simulink model "SwarmSystem"  (R2022b)
settings: Solver=VariableStepAuto  StartTime=0.0  StopTime=10.0  RelTol=1e-3
values from neighbouring files (symbols this model uses):
  dt = 0.01    [init_params.m]
  initial_state_x0 = Simulink.Parameter(initial_state_x0)    [init_params.m]    (also in single_model_verification_script.m = [W0; R0; dP0; P0]; team_model_conf_comp_script.m = [W0; R0; dP0; P0]; team_model_tethered_tilt.m = [W0; R0; dP0; P0]; team_model_tracking_script.m = [W0; R0; dP0; P0])
undefined symbols (not defined in the file or in its folder): drone_params, env_params
libraries: dspindex x15, aerolibanim x1
(part 4 of 4)

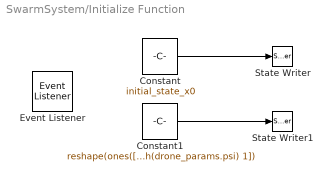
== system SwarmSystem/Initialize Function ==
  Constant : Constant  Value=initial_state_x0  VectorParams1D=off
  Constant1 : Constant  Value=reshape(ones([1 length(drone_params.psi)]) .* [0 0 0 0 1 1]', [6*length(drone_params.psi) 1])  VectorParams1D=off
  Event Listener : EventListener  DisableCoverage=on  EventName=reset
  State Writer : StateWriter  StateOwnerBlock=../../DroneState
  State Writer1 : StateWriter  StateOwnerBlock=../../InternalState
  wires:
  Constant/1 -> State Writer/1
  Constant1/1 -> State Writer1/1

== matlab function SwarmSystem/MATLAB Function3 ==
  data: R input; eulers output
function eulers = rotm2euler(R)
    psi = atan2(-R(1, 2), R(2, 2));    
    phi = atan2(R(3, 2), sqrt(abs(1-R(3, 2).^2)));
    theta = atan2(-R(3, 1), R(3, 3));
    eulers = [psi phi theta]';
end

== matlab function SwarmSystem/MATLAB Function5 ==
  data: zo input; drone_params parameter; vec output; env_params parameter
function vec = actuator_mixing(zo, drone_params, env_params)
    %% Parameters
    g = env_params.g; % gravity
    rho = env_params.rho; % kg/m3
    prop_d = env_params.prop_d; % 8 inch = 20.3 cm
    
    CT_u = env_params.CT_u; % upper propeller thrust coefficient
    CT_l = env_params.CT_l; % lower propeller thrust coefficient
    CP_u = env_params.CP_u; % upper propeller drag coefficient
    CP_l = env_params.CP_l; % lower propeller drag coefficient

    pos = drone_params.pos;
    psi = drone_params.psi;
    n = length(psi);

    Tf = zeros([n 1]);
    eta_x = zeros([n 1]);
    eta_y = zeros([n 1]);

    beta_allo = [CT_u CT_l; prop_d * CP_u -prop_d * CP_l];
    P_prop = rho * prop_d^4 * beta_allo;

    for i = 1:n
        % Actuator Model
        zi = zo(4 * (i - 1) + 1 : 4 * i);
        TfTdi = P_prop * zi(3:4, 1).^2;
        Tf(i) = TfTdi(1);
        eta_x(i) = zi(1);
        eta_y(i) = zi(2);
    end

    M = get_M(n, psi, pos);
    fi = get_f(eta_x, eta_y, Tf);
    vec = M * fi;
end

== matlab function SwarmSystem/MATLAB Function6 ==
  data: zo input; drone_params parameter; vec output; env_params parameter
function vec = actuator_mixing(zo, drone_params, env_params)
    %% Parameters
    g = env_params.g; % gravity
    rho = env_params.rho; % kg/m3
    prop_d = env_params.prop_d; % 8 inch = 20.3 cm
    
    CT_u = env_params.CT_u; % upper propeller thrust coefficient
    CT_l = env_params.CT_l; % lower propeller thrust coefficient
    CP_u = env_params.CP_u; % upper propeller drag coefficient
    CP_l = env_params.CP_l; % lower propeller drag coefficient

    pos = drone_params.pos;
    psi = drone_params.psi;
    n = length(psi);

    Tf = zeros([n 1]);
    eta_x = zeros([n 1]);
    eta_y = zeros([n 1]);

    beta_allo = [CT_u CT_l; prop_d * CP_u -prop_d * CP_l];
    P_prop = rho * prop_d^4 * beta_allo;

    for i = 1:n
        % Actuator Model
        zi = zo(4 * (i - 1) + 1 : 4 * i);
        TfTdi = P_prop * zi(3:4, 1).^2;
        Tf(i) = TfTdi(1);
        eta_x(i) = zi(1);
        eta_y(i) = zi(2);
    end

    M = get_M(n, psi, pos);
    fi = get_f(eta_x, eta_y, Tf);
    vec = M * fi;
end

== matlab function SwarmSystem/Actuator Compensator ==
  settings: updateMethod=DISCRETE  sampleTime=dt
  data: z input; z_d input; z_dc output; drone_params parameter; dt parameter
function z_dc = acutator_compensator(z, z_d, drone_params, dt)
    psi = drone_params.psi;
    n = length(psi);    
    
    mKp = drone_params.mKp; % Servo motor gain
    mKd = drone_params.mKd; % Servo motor gain
    pKp = drone_params.pKp; % BLDC motor gain

    sigma_x = drone_params.sigma_a;
    sigma_y = drone_params.sigma_b;
    z_dc = opt_compensator(n, z, z_d, sigma_x, sigma_y);
    %z_dc = compensator(n, z, z_d, dt, mKp, mKd, sigma_x, sigma_y);
end

function z_dc = opt_compensator(n, z, z_d, sigma_x, sigma_y)
    z_dc = z_d;
    for i=1:n
        zi = z(6*(i-1)+1 : 6*i);
        x_zi = [1 0 0 0 0 0; 0 0 1 0 0 0] * zi;
        v_zi = [0 1 0 0 0 0; 0 0 0 1 0 0] * zi;

        z_di = z_d(4*(i-1)+1 : 4*(i-1)+2);
        %z_dcr = -14.3636 * (x_zi-z_di) - 0.3070 * (v_zi-0) + 0.6924 * z_di;
        z_dcr = -28.0209 * (x_zi-z_di) -0.5379 * (v_zi-0) + 0.9971 * z_di;
        %z_dcr = -17.3915 * (x_zi-z_di) -0.4492 * (v_zi-0) + 0.8054 * z_di;
        %z_dcr = -11.8288 * (x_zi-z_di) -0.4958 * (v_zi-0) + 0.4905 * z_di;
        
        z_dcr(1) = min(sigma_x, max(-sigma_x, z_dcr(1)));
        z_dcr(2) = min(sigma_y, max(-sigma_y, z_dcr(2)));

        z_dc(4*(i-1)+1 : 4*(i-1)+2) = z_dcr;
    end
end

function z_dc = compensator(n, z, z_d, dt, mKp, mKd, sigma_x, sigma_y)
    w_n = sqrt(mKp);
    zeta = mKd / (2 * w_n);
    k = mKp;

    w_d = w_n * sqrt(1 - zeta^2);
    sigma = -zeta * w_n;

    C1 = (w_n / w_d) * exp(sigma * dt) * sin(w_d * dt + atan(w_d / -sigma));
    C2 = (exp(sigma * dt) / w_d) * sin(w_d * dt);
    C3 = (k / w_d) * (w_d + exp(sigma * dt) * (sigma*sin(w_d*dt) - w_d*cos(w_d*dt))) / w_n^2;

    z_dc = z_d;
    %return
    
    for i=1:n
        zi = z(6*(i-1)+1 : 6*i);
        x_zi = [1 0 0 0 0 0; 0 0 1 0 0 0] * zi;
        v_zi = [0 1 0 0 0 0; 0 0 0 1 0 0] * zi;

        z_di = z_d(4*(i-1)+1 : 4*(i-1)+2);
        delta_z_di = z_di - x_zi;

        M = (delta_z_di + (1-C3-C1)*x_zi - C2*v_zi) ./ (C3 * delta_z_di);
        z_dcr = x_zi + delta_z_di .* M;
        
        z_dcr(1) = min(sigma_x, max(-sigma_x, z_dcr(1)));
        z_dcr(2) = min(sigma_y, max(-sigma_y, z_dcr(2)));

        z_dc(4*(i-1)+1 : 4*(i-1)+2) = z_dcr;
    end
end

== matlab function SwarmSystem/MATLAB Function7 ==
  data: u input; alignment output; u_d input; error output
function [alignment, error] = metrices(u, u_d)
    error = norm(u_d - u) / norm(u_d);
    alignment = u' * u_d / (norm(u_d) * norm(u));
end

== matlab function SwarmSystem/MATLAB Function8 ==
  data: u input; alignment output; u_d input; error output
function [alignment, error] = metrices(u, u_d)
    error = norm(u_d - u) / norm(u_d);
    alignment = u' * u_d / (norm(u_d) * norm(u));
end

== matlab function SwarmSystem/Full-Pose Controller ==
  settings: updateMethod=DISCRETE  sampleTime=dt
  data: x_r input; u_d output size=[6 1]; R_r input; x input; env_params parameter; drone_params parameter; R_d output
function [u_d, R_d] = full_pose_controller(x_r, R_r, x, env_params, drone_params)
    m = drone_params.m; % Mass, Kg
    g = env_params.g;
    I_b = drone_params.I_b; % Leverage length from c.p. to c.g.
    
    % States
    p = x(16:18);
    v = x(13:15);
    R = reshape(x(4:12), [3 3]); % 3x3
    w = x(1:3);
    
    % Gain
    Kp = diag([1 1 1]) * 0.2 * 10;
    Kd = diag([1 1 1]) * 0.5 * 10;
    Kr = diag([1 1 1]) * 3 * 10;
    Ko = diag([1 1 1]) * 1 * 10;
    
    % % Translational error
    ep = p - x_r(1:3, 1);
    ev = v - x_r(1:3, 2);
    
    f_r = m * x_r(1:3, 3) + m*[0; 0; g] + m * (- Kp * ep - Kd * ev);
    u_f = R' * f_r;
    u_f = force_sat(drone_params, u_f);
    
    [R_d, theta] = calc_R_d(drone_params, f_r, R_r);
    %R_d = R_r;
    % w_d = vee(R_d' * d_R_d);
    
    % Attitude error
    eRx = 0.5 * (R_d' * R - R' * R_d);
    eR = vee(eRx);
    % eOmega = w - R' * R_d * w_d;
    eOmega = w;
    
    u_tau = cross(w, I_b * w) + I_b * ( - Kr * eR - Ko * eOmega);
    u_d = [u_f; u_tau];
end

function u_sat = force_sat(drone_params, u)
    psi = drone_params.psi;
    sigma_a = drone_params.sigma_a;
    f_max = drone_params.f_max;
    n = length(psi);

    n_x = sum(psi == 0);
    n_y = n - n_x;

    a = n_x * f_max + (n_y ~= 0) * u(3) * tan(sigma_a);
    b = n_y * f_max + (n_x ~= 0) * u(3) * tan(sigma_a);
    t = (a * b) / sqrt(u(1)^2 * b^2 + u(2)^2 * a^2);

    % Directional saturation
    u_sat = u;
    if t < 1
        u_sat(1:2) = t * u(1:2);
    end

    % Magnitude saturation
    roof_lim = n * drone_params.f_max;
    scale = norm(u_sat(1:3)) / roof_lim;
    if scale > 1
        u_sat(1:3) = u_sat(1:3) / scale;
    end
end

function [R_d, theta] = calc_R_d(drone_params, f_r, R_r)
    b1r = R_r(:, 1);
    b2r = R_r(:, 2);
    b3r = R_r(:, 3);
    [theta] = ctrl_sat_square_bisection(drone_params, 20, b1r, b3r, f_r);

    k = cross(b3r, f_r) / norm(cross(b3r, f_r));
    nb3 = rot_vec_by_theta(b3r, k, theta);
    nb2 = cross(nb3, b1r) / norm(cross(nb3, b1r));
    nb1 = cross(nb2, nb3);
    R_d = [nb1 nb2 nb3];
end

function [theta] = ctrl_sat_square_bisection(drone_params, n, b1r, b3r, f_r)
    %sigma_a = conf('sigma_a');
    b2r = cross(b3r, b1r);
    theta_max = acos(b3r' * f_r / norm(f_r));
    % theta_max = asin(norm(cross(b3r, f_r)) / norm(f_r));
    theta = theta_max / 2;
    % abs(f_r' * b2r)
    % f_r' * b3r * tan(sigma_a)
    % if abs(f_r' * b2r) > f_r' * b3r * tan(sigma_a)
    if ~is_attainable(drone_params, b1r, b2r, b3r, f_r)
        k = cross(b3r, f_r) / norm(cross(b3r, f_r));
        for i=1:n
            b3 = rot_vec_by_theta(b3r, k, theta);
            b2 = cross(b3, b1r) / norm(cross(b3, b1r));
            b1 = cross(b2, b3);
            % if abs(f_r' * b2) < f_r' * b3 * tan(sigma_a)
            if is_attainable(drone_params, b1, b2, b3, f_r)
                theta = theta - 0.5 * theta_max / (2^i);
            else
                theta = theta + 0.5 * theta_max / (2^i);
            end
            % fprintf("%d: %.4f\n", i, theta)
        end
    else
        theta = 0;
    end
end

function out = rot_vec_by_theta(vec, rot_axis, theta)
    out = vec * cos(theta) + cross(rot_axis, vec) * sin(theta) + rot_axis * (rot_axis' * vec) * (1 - cos(theta));
end

function feasible = is_attainable(drone_params, b1, b2, b3, f_r)
    feasible = elliptic_cone(drone_params, b1, b2, b3, f_r);
    % feasible = pie(conf, b1, b2, b3, f_r);
end

function feasible = elliptic_cone(drone_params, b1, b2, b3, f_r)
    n = length(drone_params.psi);
    f_max = drone_params.f_max;
    sigma_a = drone_params.sigma_a;
    sigma_b = drone_params.sigma_b;

    n_x = sum(drone_params.psi == 0);
    n_y = n - n_x;

    z = f_r' * b3;
    c_x = fun_g(n_x, sigma_b, z, f_max) + fun_g(n_y, sigma_a, z, f_max);
    c_y = fun_g(n_x, sigma_a, z, f_max) + fun_g(n_y, sigma_b, z, f_max);

    feasible = (z > 0) & (((f_r' * b1 / c_x)^2 + (f_r' * b2 / c_y)^2) <= 1);
end

function gk = fun_g(n_k, sigma_k_bar, z, f_max)
    if (sigma_k_bar >= pi / 2)
        gk = n_k * f_max;
    else
        gk = (n_k > 0) * z * tan(sigma_k_bar);
    end
end

== matlab function SwarmSystem/SwarmModel ==
  data: x input; z input; dxdt output; z_d input; dzdt output; env_params parameter; drone_params parameter
function [dxdt, dzdt] = swarm_model(x, z, z_d, env_params, drone_params)
    %% Parameters
    g = env_params.g; % gravity
    rho = env_params.rho; % kg/m3
    prop_d = env_params.prop_d; % 8 inch = 20.3 cm
    
    CT_u = env_params.CT_u; % upper propeller thrust coefficient
    CT_l = env_params.CT_l; % lower propeller thrust coefficient
    CP_u = env_params.CP_u; % upper propeller drag coefficient
    CP_l = env_params.CP_l; % lower propeller drag coefficient
    
    mKp = drone_params.mKp; % Servo motor gain
    mKd = drone_params.mKd; % Servo motor gain
    pKp = drone_params.pKp; % BLDC motor gain
    
    % Bounds
    sigma_x = drone_params.sigma_a;
    sigma_y = drone_params.sigma_b;
    r_sigma_x = drone_params.r_sigma_a;
    r_sigma_y = drone_params.r_sigma_b;
    
    % TODO:
    sigma_w0 = drone_params.sigma_w0;
    sigma_w = drone_params.prop_max;
    r_sigma_w = drone_params.r_sigma_w;
    r_f = drone_params.r_f;
    
    % Drone
    m = drone_params.m;
    I_b = drone_params.I_b; % Body Inertial
    
    pos = drone_params.pos;
    psi = drone_params.psi;
    n = length(psi);
    
    % State 
    W = x(1:3);
    I_R_B = reshape(x(4:12), [3 3]); % 3x3
    dP = x(13:15);
    P = x(16:18);
    
    dzdt = zeros([6 * n 1]);
    Tf = zeros([n 1]);
    eta_x = zeros([n 1]);
    eta_y = zeros([n 1]);

    
    %% Actuator Model
    [A_z, B_z, C_z] = gen_actuator_model(mKp, mKd, pKp);
    % Propeller model
    beta_allo = [CT_u CT_l; prop_d * CP_u -prop_d * CP_l];
    P_prop = rho * prop_d^4 * beta_allo;
    
    for i = 1:n
        % Actuator Model
        zi = z(6 * (i - 1) + 1 : 6 * i);
        z_di = z_d(4*(i-1)+1 : 4*i);

        z_low = [-sigma_x; -r_sigma_x; -sigma_y; -r_sigma_y; sigma_w0; sigma_w0];
        z_upp = [ sigma_x;  r_sigma_x;  sigma_y;  r_sigma_y;  sigma_w(1);  sigma_w(2)];
        
        % Saturation
        %z_low = [-sigma_x; -r_sigma_x; -sigma_y; -r_sigma_y; sigma_w0; -r_sigma_w];
        %z_upp = [ sigma_x;  r_sigma_x;  sigma_y;  r_sigma_y;  sigma_w;  r_sigma_w];
        zi = min(z_upp, max(z_low, zi));
        dzdti = A_z * zi + B_z * z_di;

        %r_prop_max = sqrt(inv(beta_allo) / (rho * prop_d^4)) * [r_f / (2 * sqrt(abs(Tf_d(i)))); 0];
        r_prop_max = r_sigma_w;
        dz_low = [-r_sigma_x; -inf; -r_sigma_x; -inf; -r_prop_max; -r_prop_max];
        dz_upp = [ r_sigma_x;  inf;  r_sigma_x;  inf;  r_prop_max;  r_prop_max];
        dzdti = min(dz_upp, max(dz_low, dzdti));
        reaching_bound_x = ((zi(1) < -sigma_x) && (dzdti(1) < 0)) || ((zi(1) > sigma_x) && (dzdti(1) > 0));
        reaching_bound_y = ((zi(3) < -sigma_y) && (dzdti(3) < 0)) || ((zi(3) > sigma_y) && (dzdti(3) > 0));
        reaching_bound_w = ((zi(5:6) <= 0) & (dzdti(5:6) <= 0)) | ((zi(5:6) >= sigma_w) & (dzdti(5:6) >= 0));
        dzdti(1) = (~reaching_bound_x) * dzdti(1);
        dzdti(3) = (~reaching_bound_y) * dzdti(3);
        dzdti(5:6) = (~reaching_bound_w) .* dzdti(5:6);

        %dzdt(6 * (i - 1) + 1 : 6 * i) = A_z * zi + B_z * z_d;
        dzdt(6 * (i - 1) + 1 : 6 * i) = dzdti;
    
        zio = C_z * zi;
        TfTdi = P_prop * zio(3:4, 1).^2;
        Tf(i) = TfTdi(1);
        eta_x(i) = zio(1);
        eta_y(i) = zio(2);
    end
    
    u = full_dof_mixing(pos, psi, eta_x, eta_y, Tf);
    
    % Translational
    I_thrust = I_R_B * u(1:3);
    ddP = ([0; 0; -m * g] + I_thrust) / m;
    
    % Rotational
    B_M = -cross(W, I_b * W) + u(4:6);
    dW = I_b \ B_M;
    dQ = reshape(I_R_B * skew(W), [9 1]);

dxdt = [dW; dQ; ddP; dP];
end

function [A_z, B_z, C_z] = gen_actuator_model(mKp, mKd, pKp)
A_z = [   0    1    0    0    0    0;
       -mKp -mKd    0    0    0    0;
          0    0    0    1    0    0;
          0    0 -mKp -mKd    0    0;
          0    0    0    0 -pKp    0;
          0    0    0    0    0 -pKp];
B_z = [   0    0    0    0;
        mKp    0    0    0;
          0    0    0    0;
          0  mKp    0    0;
          0    0  pKp    0;
          0    0    0  pKp];
C_z = [1 0 0 0 0 0;
       0 0 1 0 0 0;
       0 0 0 0 1 0;
       0 0 0 0 0 1];
end

function vec = full_dof_mixing(P, psi, a, b, tf)
    n = length(psi);
    M = get_M(n, psi, P);
    fi = get_f(a, b, tf);
    vec = M * fi;
end

== matlab function SwarmSystem/Control Allocation ==
  settings: updateMethod=DISCRETE  sampleTime=dt
  data: Tf_d output size=[9 1]; u_d input; eta_xd output; eta_yd output; z input; drone_params parameter; env_params parameter; dt parameter; N_esp output; incre output; packed_meta output; packed_detail output; packed_tw output; packed_intersections output; validness output; sat_order output
function [Tf_d, eta_xd, eta_yd, N_esp, incre, packed_meta, packed_detail, packed_tw, packed_intersections, validness, sat_order] = ControlAllocation(u_d, z, drone_params, env_params, dt)
    sigma_x = drone_params.sigma_a;
    sigma_y = drone_params.sigma_b;
    f_max = drone_params.f_max;

%     [Tf_d, eta_xd, eta_yd] = moore_penrose_allocator(env_params, drone_params, u_d, z, dt);
%     N_esp = 0; incre = 0; packed_meta = 0; validness = 0;
%     packed_meta=0; packed_detail=0; packed_tw=0; packed_intersections=0; sat_order=0;
    [Tf_d, eta_xd, eta_yd, N_esp, incre, packed_meta, packed_detail, packed_tw, packed_intersections, validness, sat_order] = redistributed_nonlinear_allocator(env_params, drone_params, u_d, z, dt);
    %[Tf_d, eta_xd, eta_yd] = allocator_interior_point(drone_params, u_d, z);

    Tf_d = min(f_max, max(0, Tf_d));
    eta_xd = min(sigma_x, max(-sigma_x, eta_xd));
    eta_yd = min(sigma_y, max(-sigma_y, eta_yd));
end

%%%%%%%%%%%%%%%%%%%%%%%%%%%%%%%%%%%%%%%%%%%%%%%%%%%%%%%%%%%%%%%%%%%%%%%%%%%

function [Tf_d, eta_xd, eta_yd] = allocator_interior_point(drone_params, u_d, z)
    % Configurations
    P = drone_params.pos;
    psi = drone_params.psi;
    sigma_x = drone_params.sigma_a;
    sigma_y = drone_params.sigma_b;
    f_max = drone_params.f_max;

    n = length(psi);
    W = eye(3*n);
    M = get_M(n, psi, P);

    x0 = zeros(3*n, 1);
    %Tf_d = zeros(n, 1);
    %u0 = get_f(a0, b0, f0);
%     u0 = [];
% 
    for i = 1:n
        x0(i * 3) = 10;
    end

    % x = fmincon(fun,    x0,  A,  b,Aeq,beq, lb, ub, nonlcon)
    options = optimoptions(@fmincon, 'Algorithm', 'sqp', 'Display', 'off');
    Fi = fmincon(@(x)costfun(n, x, M, u_d), x0, [], [], [], [], [], [], @(x)mycon(n, x, f_max, sigma_x, sigma_y), options);
    [Tf_d, eta_xd, eta_yd] = inverse_input(n, Fi);


    % constrain on angles
    function [c, ceq] = mycon(n, xx, f_max, sigma_x, sigma_y)
        [Fc, ac, bc] = inverse_input(n, xx);
        c = [-Fc;
            Fc - f_max;
            -sigma_x - ac;
            ac - sigma_x;
            -sigma_y - bc;
            bc - sigma_y];
        ceq = [];
    end
    
    function y = costfun(n, xx, M, u_d)
        Fi_f = reshape(xx, [3, n]);
        F_f = sqrt(sum(Fi_f.^2, 1))';
        y_f = F_f' * F_f;
    
        y = sum((M*xx - u_d).^2) + y_f;
        
        % y = F' * W * F + 0.01 * (x - u0)' * eye(30) * (x - u0);
    end
end

%%%%%%%%%%%%%%%%%%%%%%%%%%%%%%%%%%%%%%%%%%%%%%%%%%%%%%%%%%%%%%%%%%%%%%%%%%%

function [Tf_d, eta_xd, eta_yd, N_esp, c, packed_meta, packed_detail, packed_tw, packed_intersections, validness, sat_order] = redistributed_nonlinear_allocator(env_params, drone_params, u_d, z, dt)
    rate_cons = true;
    % Configurations
    P = drone_params.pos;
    psi = drone_params.psi;
    f_max = drone_params.f_max;
    pinv_tol = 0.0001;

    n = length(psi);
    M = get_M(n, psi, P);

    % Initialization
    N_esp = ones([n 1]);
    M_esp = M;
    c = 0;

    packed_detail = zeros([n, 3*n]);
    packed_tw = zeros([n, n, 3]);
    packed_intersections = zeros([n, n, 3, 3]);

    if rate_cons
        [Tf0, eta_x0, eta_y0] = z2raw(n, z, env_params);
        [lower_x, upper_x, lower_y, upper_y] = solve_upper_lower_bounds(drone_params, dt, Tf0, eta_x0, eta_y0);
        packed_meta = [lower_x upper_x lower_y upper_y];
        %Tf0(Tf0 > f_max) = f_max;  % scaling down a bit
        u0 = get_f(eta_x0, eta_y0, Tf0);
        %validness = (lower_x <= eta_x0) & (eta_x0 <= upper_x) & (lower_y <= eta_y0) & (eta_y0 <= upper_y);
    else
        sigma_x = drone_params.sigma_a;
        sigma_y = drone_params.sigma_b;
        lower_x = -sigma_x * ones([n 1]);
        upper_x = sigma_x * ones([n 1]); 
        lower_y = -sigma_y * ones([n 1]);
        upper_y = sigma_y * ones([n 1]);
        u0 = get_f(zeros([n 1]), zeros([n 1]), ones([n 1]));
    end

    t0 = M * u0;
    t_delta = u_d - t0;
    idx = 1;

    sat_order = zeros([n, 1]);

    % Iteration
    while (c < 1) && (rank(M_esp) >= 6)
        % Calculate
        M_esp = M * kron(diag(N_esp), eye(3)); % masking
        M_esp_dag = pinv(M_esp, pinv_tol);
        u_delta = M_esp_dag * t_delta;

        %[d_max, i_star, N_esp, ti, tw] = calc_nearest_c2(N_esp, u0, u0 + u_delta, sigma_x, sigma_y, f_max);
        [d_max, i_star, N_esp, ti, tw, txn, txp] = calc_nearest_c2(N_esp, u0, u0 + u_delta, lower_x, upper_x, lower_y, upper_y, f_max);

        if d_max == inf
            idx = idx + 1;
            break;
        end

        % Update marked set
        for l=1:length(i_star)
            N_esp(i_star(l)) = 0;
            sat_order(idx) = i_star(l);
        end
        %N_esp(i_star) = 0;
        d = d_max;

        if d_max > 1 - c
            d = 1 - c;
        end


        u0 = u0 + d * u_delta;
        c = c + d; 

        packed_detail(idx, :) = u0';
        packed_tw(idx, :, :) = tw;
        u0_xyz = reshape(u0, [3, n]);
        u_delta_xyz = reshape(u_delta, [3, n]);
        for k = 1:n
            packed_intersections(idx, k, 1, :) = (u0_xyz(:, k) + u_delta_xyz(:, k) * tw(k, 2))';
            packed_intersections(idx, k, 2, :) = (u0_xyz(:, k) + u_delta_xyz(:, k) * txn(k))';
            packed_intersections(idx, k, 3, :) = (u0_xyz(:, k) + u_delta_xyz(:, k) * txp(k))';
        end
        
        idx = idx + 1;
    end
    [Tf_d, eta_xd, eta_yd] = inverse_input(n, u0);

    % Check for validness
    %validness = (lower_x <= eta_xd) & (eta_xd <= upper_x) & (lower_y <= eta_yd) & (eta_yd <= upper_y);
    validness = sqrt((lower_x > eta_xd) .* (lower_x - eta_xd).^2 + ...  
                     (eta_xd > upper_x) .* (eta_xd - upper_x).^2 + ... 
                     (lower_y > eta_yd) .* (lower_y - eta_yd).^2 + ... 
                     (eta_yd > upper_y) .* (eta_yd - upper_y).^2);
%     validness = (lower_x > eta_x0) .* (lower_x - eta_x0).^2 + ...  
%                 (eta_x0 > upper_x) .* (eta_x0 - upper_x).^2 + ... 
%                 (lower_y > eta_y0) .* (lower_y - eta_y0).^2 + ... 
%                 (eta_y0 > upper_y) .* (eta_y0 - upper_y).^2;
    %alignment = (u_d(4:6)' * (M(4:6, :) * u0)) / (norm(u_d(4:6)) * norm(M(4:6, :) * u0));
    %validness = alignment;
end

function [c_star, i_star, N_esp, ti, tw, txn, txp] = calc_nearest_c2(N_esp, u0, ud, lower_x, upper_x, lower_y, upper_y, f_max)
%function [c_star, i_star, N_esp, ti, tw] = calc_nearest_c2(N_esp, u0, ud, sigma_a, sigma_b, f_max)
    % u0: allocation result in previous step
    % ud: temporary target

    % u is 3n x 1 column vector
    % u_xyz is 3 x n matrix
    % v is alias for u / tan
    n = length(N_esp);
    u_xyz = reshape(u0, [3 n]);
    u_delta = ud - u0;
    u_delta_xyz = reshape(u_delta, [3, n]);
    % u_delta_xyz(:, ~N_esp) = 0; % disabled actuators

    % Determine direction
    [f0, a0, b0] = inverse_input(n, u0);
    [f1, a1, b1] = inverse_input(n, ud);
    % norm(get_f(a1, b1, f1) - ud)
    a_s = lower_x;
    b_s = lower_y;
    a_s(a1 - a0 > 0) = upper_x(a1 - a0 > 0);
    b_s(b1 - b0 > 0) = upper_y(b1 - b0 > 0);
%     [df0, da0, db0] = inverse_input(n, ud-u0);
%     % norm(get_f(a1, b1, f1) - ud)
%     a_s = lower_x;
%     b_s = lower_y;
%     a_s(da0 > 0) = upper_x(da0 > 0);
%     b_s(db0 > 0) = upper_y(db0 > 0);

    % Finding nearest
    [tw, txn, txp] = solve_intersections(u_xyz, u_delta_xyz, a_s, b_s, f_max);

    % Checking direction of delta
    is_at_origin = norm(u_xyz(3, :)) == 0;
    [df1, da1, db1] = inverse_input(n, u_delta);
    mask_da = (lower_x <= da1) & (da1 <= upper_x); % in range
    mask_db = (lower_y <= db1) & (db1 <= upper_y); 
    t_dir = is_at_origin' & mask_da & mask_db;

    % Checking direction of delta
    tw(tw < 0) = inf;        % Not intersecting in forward direction
    ti = min(tw, [], 2);     % The nearest collision in the 3 DOFs
    ti(N_esp <= 0) = inf;    % 
    ti(t_dir > 0) = inf;

    [c_star, i_star] = min(ti); % deal with the case of multiple minimums
    i_star = find(ti == c_star);
end

function [tw, txn, txp] = solve_intersections(u_xyz, u_delta_xyz, a_s, b_s, f_max)
    % a_s: bound of a (pos / neg sigmal_a, according to the direction of delta)
    % b_s: bound of a (pos / neg sigmal_b, according to the direction of delta)
    v_delta_y = u_delta_xyz(2, :) ./ (tan(a_s)');
    v_xyz_y = u_xyz(2, :) ./ (tan(a_s)');
    v_norm = vecnorm(u_delta_xyz, 2, 1)';
    tf0 = vecnorm(u_xyz, 2, 1)';

    % y-axis
    txa = u_delta_xyz(1, :)'.^2 + u_delta_xyz(3, :)'.^2 - v_delta_y'.^2;
    txb = u_xyz(1, :)' .* u_delta_xyz(1, :)' + u_xyz(3, :)' .* u_delta_xyz(3, :)' - v_xyz_y' .* v_delta_y';
    txc = u_xyz(1, :)'.^2 + u_xyz(3, :)'.^2 - v_xyz_y'.^2;
    tx1 = (-txb - sqrt(abs(txb.^2 - txa .* txc))) ./ txa;
    tx2 = (-txb + sqrt(abs(txb.^2 - txa .* txc))) ./ txa;

    txn = tx1; % Make the txn really the smaller one
    txn(tx2 < tx1) = tx2(tx2 < tx1);
    txp = tx2; % Make the txp really the larger one
    txp(tx2 < tx1) = tx1(tx2 < tx1);
    tx = txn; % Choose the non-negative one
    tx(tx < 0) = txp(tx < 0);

%     tx = (-txb - sqrt(abs(txb.^2 - txa .* txc))) ./ txa;
%     txp = (-txb + sqrt(abs(txb.^2 - txa .* txc))) ./ txa;
%     txn = tx;
%     tx(tx < 0) = txp(tx < 0);
    
    mask_no_sol = txb.^2 - txa .* txc < 0;
    tx(mask_no_sol) = inf;

    txl = -txc ./ (2 * txb);
    mask_a_small = abs(txa) < 1e-20;
    tx(mask_a_small) = txl(mask_a_small);

    % x-axis
    ty = -(u_xyz(1, :)' - u_xyz(3, :)' .* tan(b_s)) ./ (u_delta_xyz(1, :)' - u_delta_xyz(3, :)' .* tan(b_s));
    mask_no_sol = (u_delta_xyz(1, :)' == (u_delta_xyz(3, :)' .* tan(b_s)));
    ty(mask_no_sol) = inf;

    % z-axis
%     kkb = dot(u_xyz, u_delta_xyz, 1)' ./ v_norm.^2;
%     kkc = (tf0 .* tf0 - f_max^2) ./ v_norm.^2;
%     tz = -kkb + sqrt(abs(kkb .* kkb - kkc));
    kkb = dot(u_xyz, u_delta_xyz, 1)';
    kkc = (tf0 .^ 2 - f_max^2);
    tz = (-kkb + sqrt(abs(kkb .* kkb - v_norm.^2 .* kkc))) ./ v_norm.^2;

    mask_a_small = abs(v_norm.^2) < 1e-20;
    tzl = -kkc ./ (2 * kkb);    
    tz(mask_a_small) = tzl(mask_a_small);

    mask_no_sol = kkb .^ 2 - v_norm.^2 .* kkc < 0;
    tz(mask_no_sol) = inf;
    %tz(tz<0) = 0;

%     tz = -kkb + sqrt(abs(kkb .* kkb - kkc));  
%     % the case of moving in an opposite direction
%     tzp = -kkb - sqrt(abs(kkb .* kkb - kkc));
%     tz(tz < 0) = tzp(tz < 0);
%     mask_no_sol = kkb .* kkb - kkc < 0;
%     tz(mask_no_sol) = inf;

    tw = [ty tx tz];
end

function [Tf_d, eta_xd, eta_yd] = moore_penrose_allocator(env_params, drone_params, u_d, z, dt)
    % Configurations
    P = drone_params.pos;
    psi = drone_params.psi;

    n = length(psi);
    M = get_M(n, psi, P);

    % Fi = pseudo_inverse(M) * u;
    pinv_tol = 0.0001;
    Fi = pinv(M, pinv_tol) * u_d;
    [Tf_d, eta_xd, eta_yd] = inverse_input(n, Fi);

    % Saturation
    [Tf0, eta_x0, eta_y0] = z2raw(n, z, env_params);
    [Tf_d, eta_xd, eta_yd] = saturation_with_internal_dynamic(drone_params, dt, Tf_d, eta_xd, eta_yd, Tf0, eta_x0, eta_y0);
end

function [lower_x, upper_x, lower_y, upper_y] = solve_upper_lower_bounds(drone_params, dt, Tf0, eta_x0, eta_y0)
    %% Parameters
    sigma_x = drone_params.sigma_a;
    sigma_y = drone_params.sigma_b;
    r_sigma_x = drone_params.r_sigma_a;
    r_sigma_y = drone_params.r_sigma_b;

    lower_x = max(-sigma_x, eta_x0 - r_sigma_x * dt);
    upper_x = min( sigma_x, eta_x0 + r_sigma_x * dt);

    lower_y = max(-sigma_y, eta_y0 - r_sigma_y * dt);
    upper_y = min( sigma_y, eta_y0 + r_sigma_y * dt);
end

function [Tf_d, eta_xd, eta_yd] = saturation_with_internal_dynamic(drone_params, dt, Tf, eta_x, eta_y, Tf0, eta_x0, eta_y0)
    [lower_x, upper_x, lower_y, upper_y] = solve_upper_lower_bounds(drone_params, dt, Tf0, eta_x0, eta_y0);
    eta_xd = sat(eta_x, lower_x, upper_x);
    eta_yd = sat(eta_y, lower_y, upper_y);
    Tf_d = Tf;
end

== matlab function SwarmSystem/MATLAB Function ==
  settings: updateMethod=DISCRETE  sampleTime=dt
  data: Tf_d input; z_d output; eta_xd input; eta_yd input; env_params parameter; drone_params parameter
function z_d = calc_prop_raw_command(Tf_d, eta_xd, eta_yd, env_params, drone_params)
    % Parameters
    rho = env_params.rho; % kg/m3
    prop_d = env_params.prop_d; % 8 inch = 20.3 cm

    CT_u = env_params.CT_u; % upper propeller thrust coefficient
    CT_l = env_params.CT_l; % lower propeller thrust coefficient
    CP_u = env_params.CP_u; % upper propeller drag coefficient
    CP_l = env_params.CP_l; % lower propeller drag coefficient

    sigma_x = drone_params.sigma_a;
    sigma_y = drone_params.sigma_b;
    sigma_w0 = drone_params.sigma_w0;
    sigma_w = drone_params.prop_max;

    psi = drone_params.psi;
    n = length(psi);

    % Inversing
    beta_allo = [CT_u CT_l; prop_d * CP_u -prop_d * CP_l];

    z_d = zeros([4*n 1]);
    for i=1:n
        wm_d = sqrt(beta_allo \ [Tf_d(i); 0] / (rho * prop_d^4));
        z_di = [eta_xd(i); eta_yd(i); wm_d];

        z_low = [-sigma_x; -sigma_y;   sigma_w0;    sigma_w0];
        z_upp = [ sigma_x;  sigma_y; sigma_w(1);  sigma_w(2)];
        z_d(4*(i-1)+1 : 4*i) = min(z_upp, max(z_low, z_di));
    end
end

== matlab function SwarmSystem/MATLAB Function4 ==
  data: t input; x_r output; R_r output
function [x_r, R_r] = gen_trajectory(t)
    coder.extrinsic('init_traj');
    traj_func = zeros([6 3]);
    traj_func = init_traj(t);
    traj = traj_func;
    x_r = traj(1:3, :);

    psi_d = traj(6, 1); phi_d = traj(5, 1); theta_d = traj(4, 1);
    R_r = getI_R_B(psi_d, phi_d, theta_d);
end

function I_R_B = getI_R_B(psi, phi, theta)
    I_R_B = Rz(psi) * Rx(phi) * Ry(theta);
end

== matlab function SwarmSystem/MATLAB Function1 ==
  data: R input; eulers output
function eulers = rotm2euler(R)
    psi = atan2(-R(1, 2), R(2, 2));    
    phi = atan2(R(3, 2), sqrt(abs(1-R(3, 2).^2)));
    theta = atan2(-R(3, 1), R(3, 3));
    eulers = [psi phi theta]';
end

== matlab function SwarmSystem/MATLAB Function2 ==
  data: R input; eulers output
function eulers = rotm2euler(R)
    psi = atan2(-R(1, 2), R(2, 2));    
    phi = atan2(R(3, 2), sqrt(abs(1-R(3, 2).^2)));
    theta = atan2(-R(3, 1), R(3, 3));
    eulers = [psi phi theta]';
end
